simulink model "rst_auto_reg_2"  (R2019a)
settings: Solver=VariableStepAuto  StartTime=0.0  StopTime=50  RelTol=1e-3
undefined symbols (not defined in the file): A, B, ep, T_a, Ts
libraries: dspinverses x1
settings Model: Creator=Carlos Henrique  LastModifiedBy=PICHAU
settings DataIOCC: SaveOutput=off  SaveState=on  SignalLogging=off  DSMLogging=off  ReturnWorkspaceOutputs=off
settings DebuggingCC: ArithmeticOperatorsInVariantConditions=warning

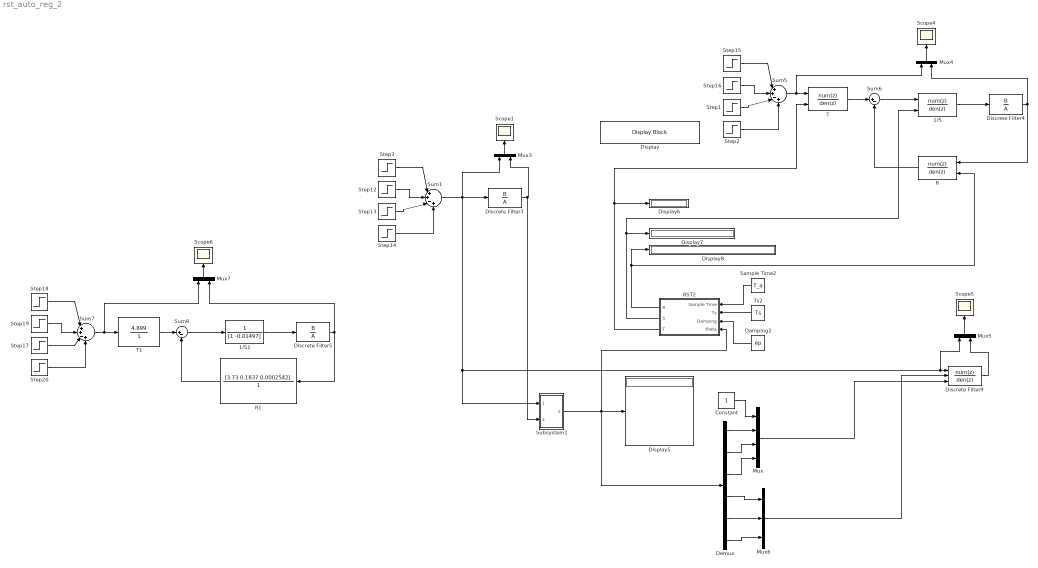
== system rst_auto_reg_2 ==
  1/S : DiscreteFilter  Numerator=1  DenominatorSource=Input port  Denominator=1  a0EqualsOne=on
      settings: InputPortMap=u0,p3
  1/S1 : DiscreteFilter  Numerator=1  Denominator=[1 -0.01497]  a0EqualsOne=on
  Constant : Constant
  Damping2 : Constant  Value=ep
  Demux : Demux  Outputs=6
  Discrete Filter3 : DiscreteFilter  Numerator=B  Denominator=A
  Discrete Filter4 : DiscreteFilter  Numerator=B  Denominator=A  SampleTime=0.1  a0EqualsOne=on
  Discrete Filter5 : DiscreteFilter  Numerator=B  Denominator=A  SampleTime=0.1  a0EqualsOne=on
  Discrete Filter9 : DiscreteFilter  NumeratorSource=Input port  Numerator=[3.317e-09 0.0355 0.02469]  DenominatorSource=Input port  Denominator=[1 -1.272 0.3317 0.0004192]  a0EqualsOne=on
      settings: InputPortMap=u0,p1,p3
  Display : DisplayBlock  LabelPosition=Hide
  Display{5..8} (4 alike) : Display
  Mux : Mux
  Mux{3..5,7} (4 alike) : Mux  Inputs=2
  Mux6 : Mux  Inputs=3
  R : DiscreteFilter  NumeratorSource=Input port  Numerator=[-620.2 131.3]  Denominator=1
      settings: InputPortMap=u0,p1
  R1 : DiscreteFilter  Numerator=[3.73 0.1837 0.0002542]  Denominator=1
  RST2 : Subsystem
  Sample Time2 : Constant  Value=T_a
  Scope{1,4..6} (4 alike) : Scope
  Step1 : Step  Time=20  After=2  SampleTime=0
  Step12 : Step  Time=10  After=3  SampleTime=0
  Step13 : Step  Time=20  After=2  SampleTime=0
  Step14 : Step  Time=30  SampleTime=0
  Step15 : Step  Time=0  SampleTime=0
  Step16 : Step  Time=10  After=3  SampleTime=0
  Step17 : Step  Time=20  After=2  SampleTime=0
  Step18 : Step  Time=0  SampleTime=0
  Step19 : Step  Time=10  After=3  SampleTime=0
  Step2 : Step  Time=30  SampleTime=0
  Step20 : Step  Time=30  SampleTime=0
  Step3 : Step  Time=0  SampleTime=0
  Subsystem1 : Subsystem
  Sum1 : Sum  Inputs=|++-+
  Sum5 : Sum  Inputs=|++-+
  Sum6 : Sum  Inputs=|+-
  Sum7 : Sum  Inputs=|++-+
  Sum8 : Sum  Inputs=|+-
  T : DiscreteFilter  NumeratorSource=Input port  Numerator=13.39  Denominator=1
      settings: InputPortMap=u0,p1
  T1 : DiscreteFilter  Numerator=4.899  Denominator=1  a0EqualsOne=on
  Ts2 : Constant  Value=Ts
  wires:
  Sum6/1 -> 1/S/1
  R/1 -> Sum6/2
  Ts2/1 -> RST2/2(Ts)
  Step2/1 -> Sum5/4
  Damping2/1 -> RST2/3(Damping)
  Sum5/1 -> Mux4/1, T/1
  T/1 -> Sum6/1
  Discrete Filter3/1 -> Mux3/2, Subsystem1/2(In2)
  Mux3/1 -> Scope1/1
  Step1/1 -> Sum5/3
  Step15/1 -> Sum5/1
  Step16/1 -> Sum5/2
  Mux4/1 -> Scope4/1
  Step3/1 -> Sum1/1
  RST2/3(T) -> T/2, Display6/1
  Sum1/1 -> Subsystem1/1(In1), Mux5/1, Discrete Filter9/1, Mux3/1, Discrete Filter3/1
  Sample Time2/1 -> RST2/1(Sample Time)
  RST2/2(S) -> 1/S/2, Display7/1
  Step12/1 -> Sum1/2
  Step14/1 -> Sum1/4
  Step13/1 -> Sum1/3
  Subsystem1/1(Out1) -> Demux/1, RST2/4(theta), Display5/1
  Mux5/1 -> Scope5/1
  Constant/1 -> Mux/1
  Demux/1 -> Mux/2
  Demux/2 -> Mux/3
  Demux/3 -> Mux/4
  Demux/4 -> Mux6/1
  Demux/5 -> Mux6/2
  Demux/6 -> Mux6/3
  Mux/1 -> Discrete Filter9/3
  Mux6/1 -> Discrete Filter9/2
  Discrete Filter9/1 -> Mux5/2
  1/S/1 -> Discrete Filter4/1
  RST2/1(R) -> R/2, Display8/1
  1/S1/1 -> Discrete Filter5/1
  Discrete Filter5/1 -> R1/1, Mux7/2
  Mux7/1 -> Scope6/1
  Step19/1 -> Sum7/2
  Step18/1 -> Sum7/1
  Step17/1 -> Sum7/3
  T1/1 -> Sum8/1
  Sum7/1 -> Mux7/1, T1/1
  Step20/1 -> Sum7/4
  R1/1 -> Sum8/2
  Sum8/1 -> 1/S1/1
  Discrete Filter4/1 -> R/1, Mux4/2

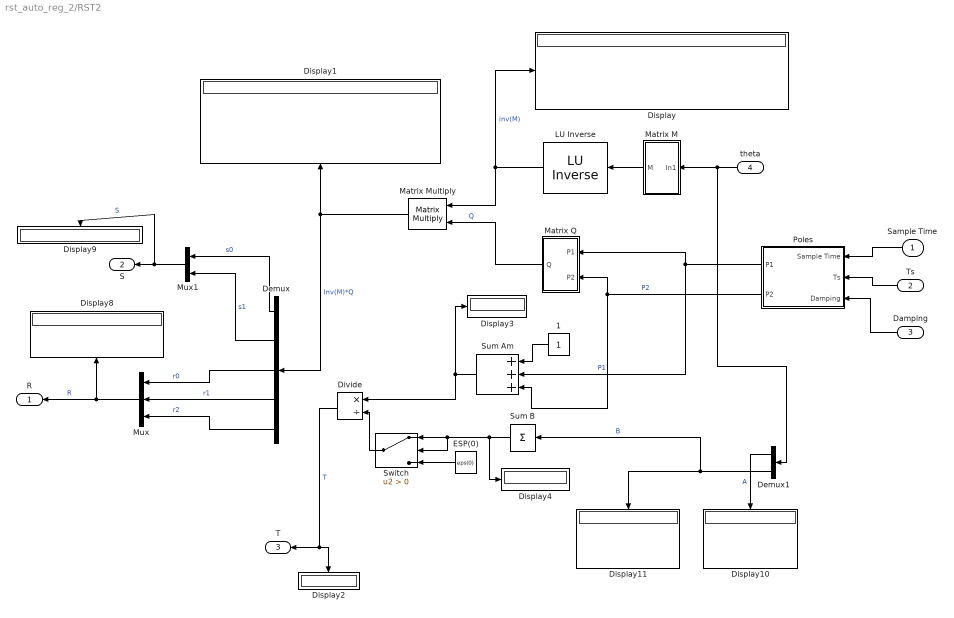
== system rst_auto_reg_2/RST2 ==
  Sample Time : Inport
  Ts : Inport  Port=2
  Damping : Inport  Port=3
  theta : Inport  Port=4
  " ESP(0)" : Constant  Value=eps(0)
  " LU Inverse" : dspinverses/ LU Inverse
      settings: SourceProductName=DSP System Toolbox
  1 : Constant
  Demux : Demux  Outputs=5
  Demux1 : Demux  Outputs=2
  Display{,1..4,8..11} (9 alike) : Display
  Divide : Product  Inputs=*/
  Matrix M : Subsystem
  Matrix Multiply : Product  Multiplication=Matrix(*)
  Matrix Q : Subsystem
  Mux : Mux  Inputs=3
  Mux1 : Mux  Inputs=2
  Poles : Subsystem
  Sum Am : Sum  Inputs=+++
  Sum B : Sum  Inputs=+
  Switch : Switch  Criteria=u2 > Threshold
  R : Outport
  S : Outport  Port=2
  T : Outport  Port=3
  wires:
  Matrix Multiply/1 -> Display1/1, Demux/1  "Inv(M)*Q"
  Sum B/1 -> Switch/2, Switch/1, Display4/1
  " LU Inverse"/1 -> Matrix Multiply/1, Display/1  "inv(M)"
  Sum Am/1 -> Divide/1, Display3/1
  Mux1/1 -> S/1, Display9/1  "S"
  Poles/2(P2) -> Matrix Q/2(P2), Sum Am/3  "P2"
  Divide/1 -> Display2/1, T/1  "T"
  Ts/1 -> Poles/2(Ts)
  Matrix Q/1(Q) -> Matrix Multiply/2  "Q"
  Damping/1 -> Poles/3(Damping)
  Sample Time/1 -> Poles/1(Sample Time)
  1/1 -> Sum Am/1
  theta/1 -> Demux1/1, Matrix M/1(In1)
  Matrix M/1(M) -> " LU Inverse"/1
  Poles/1(P1) -> Sum Am/2, Matrix Q/1(P1)  "P1"
  Demux1/2 -> Sum B/1, Display11/1  "B"
  Demux1/1 -> Display10/1  "A"
  Switch/1 -> Divide/2
  " ESP(0)"/1 -> Switch/3
  Demux/1 -> Mux1/1  "s0"
  Demux/2 -> Mux1/2  "s1"
  Mux/1 -> R/1, Display8/1  "R"
  Demux/3 -> Mux/1  "r0"
  Demux/4 -> Mux/2  "r1"
  Demux/5 -> Mux/3  "r2"

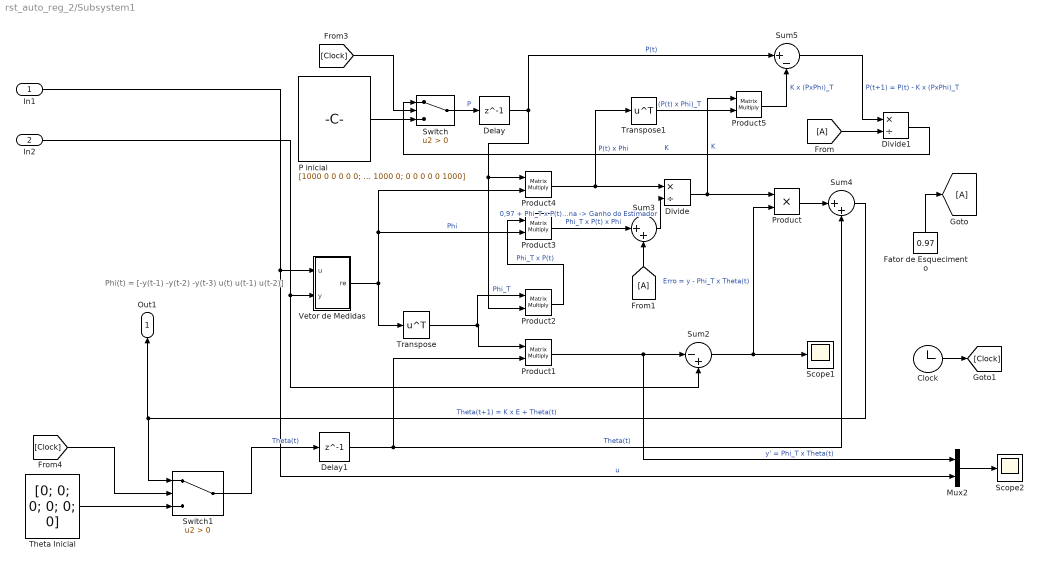
== system rst_auto_reg_2/Subsystem1 ==
  note: Phi(t) = [-y(t-1) -y(t-2) -y(t-3) u(t) u(t-1) u(t-2)]
  In1 : Inport
  In2 : Inport  Port=2
  Clock : Clock
  Delay : Delay  DelayLength=1  InitialCondition=0  SampleTime=0.1
  Delay1 : Delay  DelayLength=1  InitialCondition=0  SampleTime=0.1
  Divide : Product  Inputs=*/
  Divide1 : Product  Inputs=*/
  "Fator de Esquecimento " : Constant  Value=0.97
  Mux2 : Mux  Inputs=2
  P inicial : Constant  Value=[1000 0 0 0 0 0; 0 1000 0 0 0 0; 0 0 1000 0 0 0; 0 0 0 1000 0 0; 0 0 0 0 1000 0; 0 0 0 0 0 1000]
  Product : Product
  Product{1..5} (5 alike) : Product  Multiplication=Matrix(*)
  Scope1 : Scope
  Scope2 : Scope
  Sum2 : Sum  Inputs=|-+
  Sum3 : Sum  Inputs=|++
  Sum4 : Sum  Inputs=|++
  Sum5 : Sum  Inputs=|+-
  Switch : Switch  Criteria=u2 > Threshold
  Switch1 : Switch  Criteria=u2 > Threshold
  "Theta Inicial " : Constant  Value=[0; 0; 0; 0; 0; 0]
  Transpose : Math  Operator=transpose  SaturateOnIntegerOverflow=on
  Transpose1 : Math  Operator=transpose  SaturateOnIntegerOverflow=on
  "Vetor de Medidas " : Subsystem
  Out1 : Outport
  wires:
  "Vetor de Medidas "/1(re) -> Transpose/1, Product4/2, Product3/2  "Phi"
  Product/1 -> Sum4/1
  In2/1 -> Sum2/2, "Vetor de Medidas "/2(y)
  "Fator de Esquecimento "/1 -> [A]
  Transpose/1 -> Product2/1, Product1/1  "Phi_T"
  Sum3/1 -> Divide/2  "0,97 + Phi_T x P(t) x Phi Vetor Coluna -> Ganho do Estimador"
  Product3/1 -> Sum3/1  "Phi_T x P(t) x Phi"
  Switch/1 -> Delay/1  "P"
  Product4/1 -> Transpose1/1, Divide/1  "P(t) x Phi"
  Delay/1 -> Product4/1, Product2/2, Sum5/1  "P(t)"
  Divide/1 -> Product5/1, Product/1  "K"
  Transpose1/1 -> Product5/2  "(P(t) x Phi)_T"
  Sum5/1 -> Divide1/1  "P(t+1) = P(t) - K x (PxPhi)_T"
  Sum2/1 -> Scope1/1, Product/2  "Erro = y - Phi_T x Theta(t)"
  Delay1/1 -> Sum4/2, Product1/2  "Theta(t)"
  Divide1/1 -> Switch/1  "K"
  "Theta Inicial "/1 -> Switch1/3
  [A] -> Divide1/2
  Product2/1 -> Product3/1  "Phi_T x P(t)"
  Clock/1 -> [Clock]
  Product1/1 -> Mux2/1, Sum2/1  "y' = Phi_T x Theta(t)"
  Product5/1 -> Sum5/2  "K x (PxPhi)_T"
  P inicial/1 -> Switch/3
  Sum4/1 -> Switch1/1, Out1/1  "Theta(t+1) = K x E + Theta(t)"
  [A] -> Sum3/2
  In1/1 -> Mux2/2, "Vetor de Medidas "/1(u)  "u"
  [Clock] -> Switch/2
  Switch1/1 -> Delay1/1  "Theta(t)"
  Mux2/1 -> Scope2/1
  [Clock] -> Switch1/2

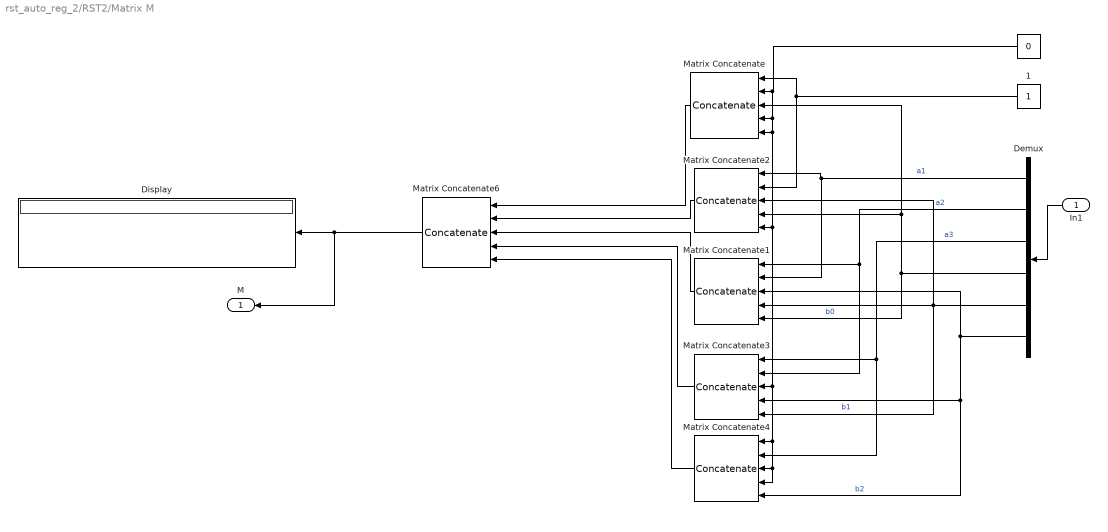
== system rst_auto_reg_2/RST2/Matrix M ==
  In1 : Inport
  " " : Constant  Value=0
  " 1" : Constant
  Demux : Demux  Outputs=6
  Display : Display
  Matrix Concatenate{,1..4} (5 alike) : Concatenate  NumInputs=5  Mode=Multidimensional array  ConcatenateDimension=2
  Matrix Concatenate6 : Concatenate  NumInputs=5  Mode=Multidimensional array
  M : Outport
  wires:
  In1/1 -> Demux/1
  Matrix Concatenate6/1 -> M/1, Display/1
  Matrix Concatenate/1 -> Matrix Concatenate6/1
  Matrix Concatenate2/1 -> Matrix Concatenate6/2
  Matrix Concatenate1/1 -> Matrix Concatenate6/3
  Matrix Concatenate3/1 -> Matrix Concatenate6/4
  " 1"/1 -> Matrix Concatenate/1, Matrix Concatenate2/2
  " "/1 -> Matrix Concatenate4/4, Matrix Concatenate4/3, Matrix Concatenate4/1, Matrix Concatenate3/3, Matrix Concatenate2/5, Matrix Concatenate/5, Matrix Concatenate/4, Matrix Concatenate/2
  Demux/4 -> Matrix Concatenate2/4, Matrix Concatenate/3, Matrix Concatenate1/5  "b0"
  Demux/1 -> Matrix Concatenate1/2, Matrix Concatenate2/1  "a1"
  Demux/5 -> Matrix Concatenate3/5, Matrix Concatenate1/4, Matrix Concatenate2/3  "b1"
  Demux/2 -> Matrix Concatenate3/2, Matrix Concatenate1/1  "a2"
  Demux/6 -> Matrix Concatenate4/5, Matrix Concatenate3/4, Matrix Concatenate1/3  "b2"
  Demux/3 -> Matrix Concatenate3/1, Matrix Concatenate4/2  "a3"
  Matrix Concatenate4/1 -> Matrix Concatenate6/5

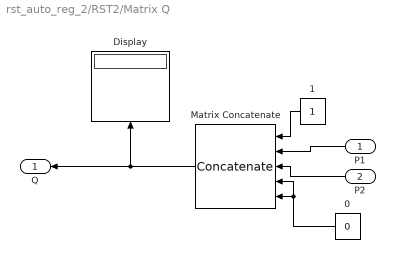
== system rst_auto_reg_2/RST2/Matrix Q ==
  P1 : Inport
  P2 : Inport  Port=2
  0 : Constant  Value=0
  1 : Constant
  Display : Display
  Matrix Concatenate : Concatenate  NumInputs=5  Mode=Multidimensional array
  Q : Outport
  wires:
  Matrix Concatenate/1 -> Q/1, Display/1
  1/1 -> Matrix Concatenate/1
  P1/1 -> Matrix Concatenate/2
  P2/1 -> Matrix Concatenate/3
  0/1 -> Matrix Concatenate/5, Matrix Concatenate/4

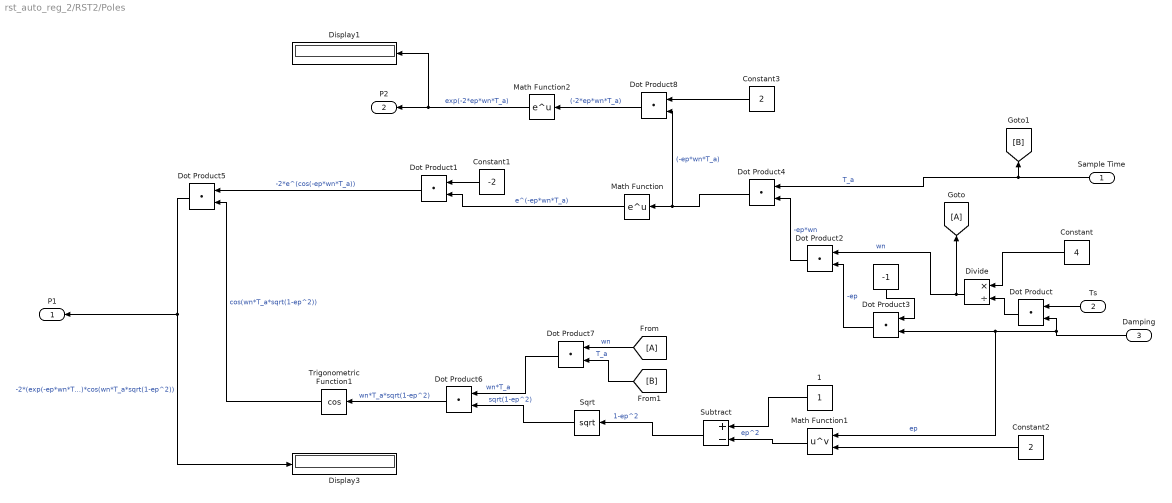
== system rst_auto_reg_2/RST2/Poles ==
  Sample Time : Inport
  Ts : Inport  Port=2
  Damping : Inport  Port=3
  " " : Constant  Value=-1
  1 : Constant
  Constant : Constant  Value=4
  Constant1 : Constant  Value=-2
  Constant2 : Constant  Value=2
  Constant3 : Constant  Value=2
  Display1 : Display
  Display3 : Display
  Divide : Product  Inputs=*/
  Dot Product{,1..8} (9 alike) : DotProduct  InputSameDT=on  OutDataTypeStr=Inherit: Inherit via internal rule
  Math Function : Math  SaturateOnIntegerOverflow=on
  Math Function1 : Math  Operator=pow  SaturateOnIntegerOverflow=on
  Math Function2 : Math  SaturateOnIntegerOverflow=on
  Sqrt : Sqrt  SaturateOnIntegerOverflow=on
  Subtract : Sum  Inputs=+-
  Trigonometric Function1 : Trigonometry  Operator=cos
  P1 : Outport
  P2 : Outport  Port=2
  wires:
  Math Function/1 -> Dot Product1/2  "e^(-ep*wn*T_a)"
  Divide/1 -> [A], Dot Product2/1  "wn"
  [A] -> Dot Product7/1  "wn"
  " "/1 -> Dot Product3/1
  Dot Product5/1 -> P1/1, Display3/1  "-2*(exp(-ep*wn*T_a))*cos(wn*T_a*sqrt(1-ep^2))"
  Trigonometric Function1/1 -> Dot Product5/2  "cos(wn*T_a*sqrt(1-ep^2))"
  Ts/1 -> Dot Product/1
  Dot Product/1 -> Divide/2
  Dot Product3/1 -> Dot Product2/2  "-ep"
  Damping/1 -> Math Function1/1, Dot Product3/2, Dot Product/2  "ep"
  Constant/1 -> Divide/1
  Dot Product7/1 -> Dot Product6/1  "wn*T_a"
  Sample Time/1 -> Dot Product4/1, [B]  "T_a"
  Math Function1/1 -> Subtract/2  "ep^2"
  Dot Product1/1 -> Dot Product5/1  "-2*e^(cos(-ep*wn*T_a))"
  Constant2/1 -> Math Function1/2
  1/1 -> Subtract/1
  Constant1/1 -> Dot Product1/1
  Dot Product2/1 -> Dot Product4/2  "-ep*wn"
  [B] -> Dot Product7/2  "T_a"
  Dot Product6/1 -> Trigonometric Function1/1  "wn*T_a*sqrt(1-ep^2)"
  Dot Product4/1 -> Dot Product8/2, Math Function/1  "(-ep*wn*T_a)"
  Sqrt/1 -> Dot Product6/2  "sqrt(1-ep^2)"
  Subtract/1 -> Sqrt/1  "1-ep^2"
  Constant3/1 -> Dot Product8/1
  Dot Product8/1 -> Math Function2/1  "(-2*ep*wn*T_a)"
  Math Function2/1 -> Display1/1, P2/1  "exp(-2*ep*wn*T_a)"

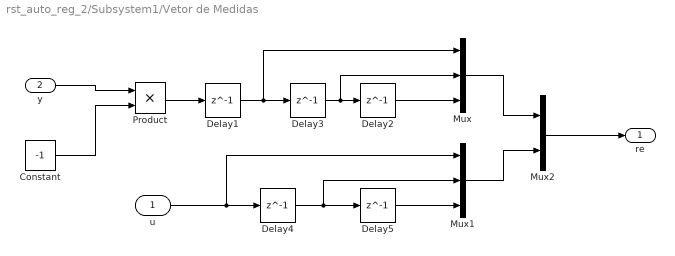
== system rst_auto_reg_2/Subsystem1/Vetor de Medidas  ==
  u : Inport
  y : Inport  Port=2
  Constant : Constant  Value=-1
  Delay{1..5} (5 alike) : Delay  DelayLength=1  InitialCondition=0  SampleTime=0.1
  Mux : Mux  Inputs=3
  Mux1 : Mux  Inputs=3
  Mux2 : Mux  Inputs=2
  Product : Product
  re : Outport
  wires:
  Delay4/1 -> Mux1/2, Delay5/1
  Delay5/1 -> Mux1/3
  Mux1/1 -> Mux2/2
  Mux/1 -> Mux2/1
  Mux2/1 -> re/1
  u/1 -> Mux1/1, Delay4/1
  Delay2/1 -> Mux/3
  y/1 -> Product/1
  Constant/1 -> Product/2
  Product/1 -> Delay1/1
  Delay3/1 -> Mux/2, Delay2/1
  Delay1/1 -> Mux/1, Delay3/1
